simulink model "onOff"  (R2013b)
settings: Solver=FixedStepDiscrete  SolverMode=SingleTasking  StartTime=0.0  StopTime=10.0  FixedStep=0.01  RelTol=1e-3
undefined symbols (not defined in the file or in its folder): JA1, JB1, JC1, nexys2iroobo_lib
libraries: xbsIndex_r4 x84
settings Model: Creator=laca  LastModifiedBy=laca
settings DebuggingCC: MultiTaskDSMMsg=warning  MultiTaskCondExecSysMsg=none  FcnCallInpInsideContextMsg=EnableAllAsWarning  StrictBusMsg=None
settings RTWCC: IncludeERTFirstTime=on

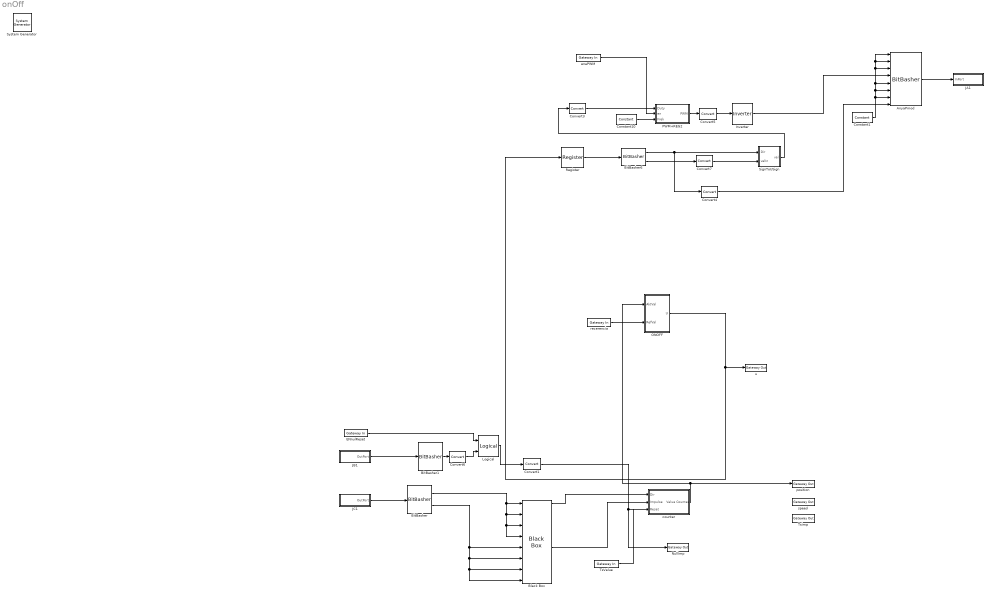
== system onOff ==
  " System Generator" : xbsIndex_r4/ System Generator  Tag=genX  xilinxfamily=spartan3e  part=xc3s1200e  speed=-4  package=fg320  synthesis_tool=XST  clock_wrapper=Clock Enables  directory=./netlist  proj_type=Project Navigator  Synth_file=XST Defaults  Impl_file=ISE Defaults  testbench=off  simulink_period=1  sysclk_period=20  dcm_input_clock_period=10  incr_netlist=off  trim_vbits=Everywhere in SubSystem  dbl_ovrd=According to Block Masks  core_generation=According to Block Masks  run_coregen=off  deprecated_control=off  eval_field=0  block_type=sysgen
  AnyaPmod : xbsIndex_r4/BitBasher  bitexpr=|  display_expr=off  sr_1=1  arith_type1=Unsigned  bin_pt1=0  sr_2=2  arith_type2=Unsigned  bin_pt2=0  sr_3=3  arith_type3=Unsigned  bin_pt3=0  sr_4=4  arith_type4=Unsigned  bin_pt4=0  dbl_ovrd=off  block_type=bitbasher
      | <!DOCTYPE HTML PUBLIC "-//W3C//DTD HTML 4.0//EN" "http://www.w3.org/TR/REC-html40/strict.dtd">
      | <html><head><meta name="qrichtext" content="1" /><style type="text/css">
      | p, li { white-space: pre-wrap; }
      | </style></head><body style=" font-family:'MS Shell Dlg 2'; font-size:8.25pt; font-weight:400; font-style:normal;">
      | <p style=" margin-top:12px; margin-bottom:12px; margin-left:0px; margin-right:0px; -qt-block-indent:0; text-indent:0px;"><span style=" font-family:'MS Shell Dlg'; font-size:8pt;">a={a8,a7,a6,a5,a4,a3,a2,a1}</span></p></body></html>
  BitBasher : xbsIndex_r4/BitBasher  bitexpr=|  display_expr=off  sr_1=1  arith_type1=Unsigned  bin_pt1=0  sr_2=2  arith_type2=Unsigned  bin_pt2=0  sr_3=3  arith_type3=Unsigned  bin_pt3=0  sr_4=4  arith_type4=Unsigned  bin_pt4=0  dbl_ovrd=off  block_type=bitbasher
      | <!DOCTYPE HTML PUBLIC "-//W3C//DTD HTML 4.0//EN" "http://www.w3.org/TR/REC-html40/strict.dtd">
      | <html><head><meta name="qrichtext" content="1" /><style type="text/css">
      | p, li { white-space: pre-wrap; }
      | </style></head><body style=" font-family:'MS Shell Dlg 2'; font-size:8.25pt; font-weight:400; font-style:normal;">
      | <p style=" margin-top:12px; margin-bottom:12px; margin-left:0px; margin-right:0px; -qt-block-indent:0; text-indent:0px;"><span style=" font-family:'MS Shell Dlg'; font-size:8pt;">A={a[0]}<br />B={a[1]}</span></p></body></html>
  BitBasher1 : xbsIndex_r4/BitBasher  bitexpr=|  display_expr=off  sr_1=1  arith_type1=Unsigned  bin_pt1=0  sr_2=2  arith_type2=Unsigned  bin_pt2=0  sr_3=3  arith_type3=Unsigned  bin_pt3=0  sr_4=4  arith_type4=Unsigned  bin_pt4=0  dbl_ovrd=off  block_type=bitbasher
      | <!DOCTYPE HTML PUBLIC "-//W3C//DTD HTML 4.0//EN" "http://www.w3.org/TR/REC-html40/strict.dtd">
      | <html><head><meta name="qrichtext" content="1" /><style type="text/css">
      | p, li { white-space: pre-wrap; }
      | </style></head><body style=" font-family:'MS Shell Dlg 2'; font-size:8.25pt; font-weight:400; font-style:normal;">
      | <p style=" margin-top:12px; margin-bottom:12px; margin-left:0px; margin-right:0px; -qt-block-indent:0; text-indent:0px;"><span style=" font-family:'MS Shell Dlg'; font-size:8pt;">Ar={ar[0]}<br /></span></p></body></html>
  BitBasher6 : xbsIndex_r4/BitBasher  bitexpr=|  display_expr=off  sr_1=1  arith_type1=Unsigned  bin_pt1=0  sr_2=2  arith_type2=Unsigned  bin_pt2=0  sr_3=3  arith_type3=Unsigned  bin_pt3=0  sr_4=4  arith_type4=Unsigned  bin_pt4=0  dbl_ovrd=off  block_type=bitbasher
      | <!DOCTYPE HTML PUBLIC "-//W3C//DTD HTML 4.0//EN" "http://www.w3.org/TR/REC-html40/strict.dtd">
      | <html><head><meta name="qrichtext" content="1" /><style type="text/css">
      | p, li { white-space: pre-wrap; }
      | </style></head><body style=" font-family:'MS Shell Dlg 2'; font-size:8.25pt; font-weight:400; font-style:normal;">
      | <p style=" margin-top:12px; margin-bottom:12px; margin-left:0px; margin-right:0px; -qt-block-indent:0; text-indent:0px;"><span style=" font-family:'MS Shell Dlg'; font-size:8pt;">dir={a[16]}<br />val={a[15:0]}</span></p></body></html>
  Black Box : xbsIndex_r4/Black Box  init_code=top_level_config  sim_method=ISE Simulator  verbose=off  block_type=blackbox2
  Constant1 : xbsIndex_r4/Constant  const=1  gui_display_data_type=Boolean  arith_type=Boolean  n_bits=16  bin_pt=0  preci_type=Single  exp_width=8  frac_width=24  explicit_period=on  period=1  equ=P=C  opselect=C  inp2=PCIN>>17  opr=+  inp1=P  carry=CIN  dbl_ovrd=off  block_type=constant
  Constant10 : xbsIndex_r4/Constant  const=65535  gui_display_data_type=Fixed-point  arith_type=Unsigned  n_bits=16  bin_pt=0  preci_type=Single  exp_width=8  frac_width=24  explicit_period=on  period=1  equ=P=C  opselect=C  inp2=PCIN>>17  opr=+  inp1=P  carry=CIN  dbl_ovrd=off  block_type=constant
  Convert1 : xbsIndex_r4/Convert  gui_display_data_type=Fixed-point  arith_type=Unsigned  n_bits=1  bin_pt=0  float_type=Single  exp_bits=8  fraction_bits=24  quantization=Truncate  overflow=Wrap  en=off  latency=0  dbl_ovrd=off  pipeline=off  block_type=convert
  Convert3 : xbsIndex_r4/Convert  gui_display_data_type=Fixed-point  arith_type=Unsigned  n_bits=16  bin_pt=0  float_type=Single  exp_bits=8  fraction_bits=24  quantization=Truncate  overflow=Wrap  en=off  latency=0  dbl_ovrd=off  pipeline=off  block_type=convert
  Convert4 : xbsIndex_r4/Convert  gui_display_data_type=Boolean  arith_type=Boolean  n_bits=17  bin_pt=0  float_type=Single  exp_bits=8  fraction_bits=24  quantization=Truncate  overflow=Wrap  en=off  latency=0  dbl_ovrd=off  pipeline=off  block_type=convert
  Convert5 : xbsIndex_r4/Convert  gui_display_data_type=Boolean  arith_type=Boolean  n_bits=17  bin_pt=0  float_type=Single  exp_bits=8  fraction_bits=24  quantization=Truncate  overflow=Wrap  en=off  latency=0  dbl_ovrd=off  pipeline=off  block_type=convert
  Convert6 : xbsIndex_r4/Convert  gui_display_data_type=Boolean  arith_type=Boolean  n_bits=17  bin_pt=0  float_type=Single  exp_bits=8  fraction_bits=24  quantization=Truncate  overflow=Wrap  en=off  latency=0  dbl_ovrd=off  pipeline=off  block_type=convert
  Convert7 : xbsIndex_r4/Convert  gui_display_data_type=Fixed-point  arith_type=Unsigned  n_bits=16  bin_pt=0  float_type=Single  exp_bits=8  fraction_bits=24  quantization=Truncate  overflow=Wrap  en=off  latency=0  dbl_ovrd=off  pipeline=off  block_type=convert
  ENnulReset : xbsIndex_r4/Gateway In  gui_display_data_type=Boolean  arith_type=Boolean  n_bits=17  bin_pt=0  preci_type=Single  exp_width=8  frac_width=24  quantization="Round  (unbiased: +/- Inf)"  overflow=Saturate  period=1  dbl_ovrd=off  timing_constraint=None  locs_specified=off  LOCs={}  UseAsADC=off  ADCChannel='1'  inherit_from_input=off  hdl_port=on  block_type=gatewayin
  Inverter : xbsIndex_r4/Inverter  en=off  latency=0  dbl_ovrd=off  block_type=inv
  JA1 : Subsystem  AncestorBlock=nexys2iroobo_lib/JA1  mask(Non-Memory-Mapped Output Port){show_out=off}
      mask prompts: show_out "Provide Output Double"
      mask help:
      | Port Name: "JA1"
      | Port Type: 8-bit Vector
      mask init:
      | [bg,fg] = xlcmap('IO',0);
      | iPos = get_param(gcb,'Position');
      | iWidth=iPos(3)-iPos(1);
      | iHeight=iPos(4)-iPos(2);
      | [logoX, logoY] = xlogo(iPos);
      | if (show_out)
      |     old = find_system(gcb, 'LookUnderMasks', 'all', 'Name', 'Terminator');
      |     if (length(old) > 0)
      |         replace_block(gcb, 'Name', 'Terminator', 'OutPort', 'noprompt');
      |         set_param([gcb '/Terminator'], 'Name', 'OutPort');
      |     end
      |     portdir = 'output';
      |     portstr = 'dbl';
      | else
      |     old = find_system(gcb, 'LookUnderMasks', 'all', 'name', 'OutPort');
      |     if (length(old) > 0)
      |         replace_block(gcb, 'Name', 'OutPort', 'Terminator', 'noprompt');
      |         set_param([gcb '/OutPort'], 'Name', 'Terminator');
      |     end
      |     portdir = 'input';
      |     portstr = '';
      | end
      settings: CopyFcn=set_param(gcb,'LinkStatus','inactive');
      mask Display:
      | patch([0 iWidth iWidth 0],[0 0 iHeight iHeight] , bg);
      | patch(logoX,logoY, fg);
      | plot([0 0 iWidth iWidth 0], [0 iHeight iHeight 0 0]);
      | port_label(portdir,1,portstr);
      | port_label('input',1,'JA1');
      | text(iWidth-10,5,'nmm');
  JB1 : Subsystem  AncestorBlock=nexys2iroobo_lib/JB1  mask(Non-Memory-Mapped Input Port){signed=off, bpt=0, show_in=off, c=0}
      mask prompts: signed "Signed  (2's comp)"; bpt "Binary Point"; show_in "Provide Input Double"; c "Constant for Simulation"
      mask help:
      | Port Name: "JB1"
      | Port Type: 8-bit Vector
      mask init:
      | [bg,fg] = xlcmap('IO',0);
      | iPos = get_param(gcb,'Position');
      | iWidth=iPos(3)-iPos(1);
      | iHeight=iPos(4)-iPos(2);
      | [logoX, logoY] = xlogo(iPos);
      | if (signed)
      |     set_param([gcb '/JB1'],'arith_type','Signed  (2''s comp)');
      | else
      |     set_param([gcb '/JB1'],'arith_type','Unsigned');
      | end
      | if (show_in)
      |     old = find_system(gcb, 'LookUnderMasks', 'all', 'Name', 'Constant');
      |     if (length(old) > 0)
      |         replace_block(gcb, 'Name', 'Constant', 'InPort', 'noprompt');
      |         set_param([gcb '/Constant'], 'Name', 'InPort');
      |     end
      |     portdir = 'input';
      |     portstr = 'dbl';
      | else
      |     old = find_system(gcb, 'LookUnderMasks', 'all', 'Name', 'InPort');
      |     if (length(old) > 0)
      |         replace_block(gcb, 'Name', 'InPort', 'Constant', 'noprompt');
      |         set_param([gcb '/InPort'], 'Name', 'Constant');
      |         set_param([gcb '/Constant'], 'Value', 'c');
      |     end
      |     portdir = 'output';
      |     portstr = '';
      | end
      settings: CopyFcn=set_param(gcb,'LinkStatus','inactive');
      mask Callback show_in:
      | mask_vis = get_param(gcb, 'MaskVisibilities');
      | if (strcmp(get_param(gcb, 'show_in'),'on'))
      |     mask_vis(4) = {'off'};
      | else
      |     mask_vis(4) = {'on'};
      | end
      | set_param(gcb, 'MaskVisibilities', mask_vis);
      mask Display:
      | patch([0 iWidth iWidth 0],[0 0 iHeight iHeight] , bg);
      | patch(logoX,logoY, fg);
      | plot([0 0 iWidth iWidth 0], [0 iHeight iHeight 0 0]);
      | port_label(portdir,1,portstr);
      | port_label('output',1,'JB1');
      | text(2,5,'nmm');
  JC1 : Subsystem  AncestorBlock=nexys2iroobo_lib/JC1  mask(Non-Memory-Mapped Input Port){signed=off, bpt=0, show_in=off, c=0}
      mask prompts: signed "Signed  (2's comp)"; bpt "Binary Point"; show_in "Provide Input Double"; c "Constant for Simulation"
      mask help:
      | Port Name: "JC1"
      | Port Type: 8-bit Vector
      mask init:
      | [bg,fg] = xlcmap('IO',0);
      | iPos = get_param(gcb,'Position');
      | iWidth=iPos(3)-iPos(1);
      | iHeight=iPos(4)-iPos(2);
      | [logoX, logoY] = xlogo(iPos);
      | if (signed)
      |     set_param([gcb '/JC1'],'arith_type','Signed  (2''s comp)');
      | else
      |     set_param([gcb '/JC1'],'arith_type','Unsigned');
      | end
      | if (show_in)
      |     old = find_system(gcb, 'LookUnderMasks', 'all', 'Name', 'Constant');
      |     if (length(old) > 0)
      |         replace_block(gcb, 'Name', 'Constant', 'InPort', 'noprompt');
      |         set_param([gcb '/Constant'], 'Name', 'InPort');
      |     end
      |     portdir = 'input';
      |     portstr = 'dbl';
      | else
      |     old = find_system(gcb, 'LookUnderMasks', 'all', 'Name', 'InPort');
      |     if (length(old) > 0)
      |         replace_block(gcb, 'Name', 'InPort', 'Constant', 'noprompt');
      |         set_param([gcb '/InPort'], 'Name', 'Constant');
      |         set_param([gcb '/Constant'], 'Value', 'c');
      |     end
      |     portdir = 'output';
      |     portstr = '';
      | end
      settings: CopyFcn=set_param(gcb,'LinkStatus','inactive');
      mask Callback show_in:
      | mask_vis = get_param(gcb, 'MaskVisibilities');
      | if (strcmp(get_param(gcb, 'show_in'),'on'))
      |     mask_vis(4) = {'off'};
      | else
      |     mask_vis(4) = {'on'};
      | end
      | set_param(gcb, 'MaskVisibilities', mask_vis);
      mask Display:
      | patch([0 iWidth iWidth 0],[0 0 iHeight iHeight] , bg);
      | patch(logoX,logoY, fg);
      | plot([0 0 iWidth iWidth 0], [0 iHeight iHeight 0 0]);
      | port_label(portdir,1,portstr);
      | port_label('output',1,'JC1');
      | text(2,5,'nmm');
  Logical : xbsIndex_r4/Logical  logical_function=AND  inputs=2  en=off  latency=0  precision=User Defined  arith_type="Signed  (2's comp)"  n_bits=1  bin_pt=0  align_bp=on  dbl_ovrd=off  block_type=logical
  NullImp : xbsIndex_r4/Gateway Out  inherit_from_input=off  hdl_port=on  timing_constraint=None  locs_specified=off  LOCs={}  UseAsDAC=off  DACChannel='1'  block_type=gatewayout
  ONOFF : Subsystem
  PWM+REG2 : Subsystem
  Register : xbsIndex_r4/Register  init=0  rst=off  en=off  dbl_ovrd=off  block_type=register
  SignToUSign : Subsystem
  TsValue : xbsIndex_r4/Gateway In  gui_display_data_type=Fixed-point  arith_type=Unsigned  n_bits=24  bin_pt=0  preci_type=Single  exp_width=8  frac_width=24  quantization="Round  (unbiased: +/- Inf)"  overflow=Saturate  period=1  dbl_ovrd=off  timing_constraint=None  locs_specified=off  LOCs={}  UseAsADC=off  ADCChannel='1'  inherit_from_input=off  hdl_port=on  block_type=gatewayin
  Tsimp : xbsIndex_r4/Gateway Out  inherit_from_input=off  hdl_port=on  timing_constraint=None  locs_specified=off  LOCs={}  UseAsDAC=off  DACChannel='1'  block_type=gatewayout
  counter : Subsystem
  enaPWM : xbsIndex_r4/Gateway In  gui_display_data_type=Boolean  arith_type=Boolean  n_bits=32  bin_pt=0  preci_type=Single  exp_width=8  frac_width=24  quantization="Round  (unbiased: +/- Inf)"  overflow=Saturate  period=1  dbl_ovrd=off  timing_constraint=None  locs_specified=off  LOCs={}  UseAsADC=off  ADCChannel='1'  inherit_from_input=off  hdl_port=on  block_type=gatewayin
  position : xbsIndex_r4/Gateway Out  inherit_from_input=off  hdl_port=on  timing_constraint=None  locs_specified=off  LOCs={}  UseAsDAC=off  DACChannel='1'  block_type=gatewayout
  recerencia : xbsIndex_r4/Gateway In  gui_display_data_type=Fixed-point  arith_type="Signed  (2's comp)"  n_bits=16  bin_pt=0  preci_type=Single  exp_width=8  frac_width=24  quantization="Round  (unbiased: +/- Inf)"  overflow=Saturate  period=1  dbl_ovrd=off  timing_constraint=None  locs_specified=off  LOCs={}  UseAsADC=off  ADCChannel='1'  inherit_from_input=off  hdl_port=on  block_type=gatewayin
  speed : xbsIndex_r4/Gateway Out  inherit_from_input=off  hdl_port=on  timing_constraint=None  locs_specified=off  LOCs={}  UseAsDAC=off  DACChannel='1'  block_type=gatewayout
  u : xbsIndex_r4/Gateway Out  inherit_from_input=off  hdl_port=on  timing_constraint=None  locs_specified=off  LOCs={}  UseAsDAC=off  DACChannel='1'  block_type=gatewayout
  wires:
  Constant10/1 -> PWM+REG2/3(Frek)
  enaPWM/1 -> PWM+REG2/2(en)
  PWM+REG2/1(PWM) -> Convert5/1
  BitBasher6/1 -> Convert4/1, SignToUSign/1(Dir)
  BitBasher6/2 -> Convert7/1
  SignToUSign/1(val) -> Convert3/1
  Inverter/1 -> AnyaPmod/4
  ONOFF/1(U) -> Register/1, u/1
  Convert3/1 -> PWM+REG2/1(Duty)
  Convert4/1 -> AnyaPmod/8
  Convert5/1 -> Inverter/1
  Convert7/1 -> SignToUSign/2(valIn)
  Register/1 -> BitBasher6/1
  AnyaPmod/1 -> JA1/1(InPort)
  Constant1/1 -> AnyaPmod/3, AnyaPmod/2, AnyaPmod/1, AnyaPmod/5, AnyaPmod/6, AnyaPmod/7
  Black Box/1 -> counter/1(Dir)
  Black Box/5 -> counter/2(Impulse)
  JC1/1(OutPort) -> BitBasher/1
  BitBasher/1 -> Black Box/4, Black Box/3, Black Box/2, Black Box/1
  BitBasher/2 -> Black Box/5, Black Box/6, Black Box/7, Black Box/8
  counter/1(Value Counter) -> ONOFF/1(AktVal), position/1
  TsValue/1 -> ?
  ? -> speed/1
  JB1/1(OutPort) -> BitBasher1/1
  Logical/1 -> Convert1/1
  ? -> Tsimp/1
  BitBasher1/1 -> Convert6/1
  ENnulReset/1 -> Logical/1
  Convert1/1 -> counter/3(Reset), NullImp/1
  Convert6/1 -> Logical/2
  recerencia/1 -> ONOFF/2(RefVal)

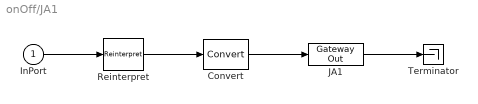
== system onOff/JA1 ==
  InPort : Inport
  Convert : xbsIndex_r4/Convert  gui_display_data_type=Fixed-point  arith_type=Unsigned  n_bits=8  bin_pt=0  float_type=Single  exp_bits=8  fraction_bits=24  quantization=Truncate  overflow=Wrap  en=off  latency=0  dbl_ovrd=off  pipeline=off  block_type=convert
  JA1 : xbsIndex_r4/Gateway Out  inherit_from_input=off  hdl_port=on  timing_constraint=None  locs_specified=on  LOCs={'M16','M14','L16','K13','M15','L17','K12','L15'}  UseAsDAC=off  DACChannel='1'  block_type=gatewayout
      settings: sginterface={'Xilinx'=>{'jtaghwcosim'=>{'non_memory_mapped_port'=>'JA1'}}}
  Reinterpret : xbsIndex_r4/Reinterpret  force_arith_type=off  arith_type=Unsigned  force_bin_pt=off  bin_pt=0  block_type=reinterpret
  Terminator : Terminator
  wires:
  JA1/1 -> Terminator/1
  Convert/1 -> JA1/1
  Reinterpret/1 -> Convert/1
  InPort/1 -> Reinterpret/1

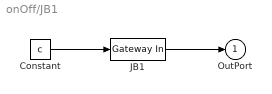
== system onOff/JB1 ==
  Constant : Constant  Value=c
  JB1 : xbsIndex_r4/Gateway In  gui_display_data_type=Fixed-point  arith_type=Unsigned  n_bits=8  bin_pt=max(0,min(bpt,8))  preci_type=Single  exp_width=8  frac_width=24  quantization="Round  (unbiased: +/- Inf)"  overflow=Saturate  period=1  dbl_ovrd=off  timing_constraint=None  locs_specified=on  LOCs={'U18','T18','R16','P17','T17','R15','R18','M13'}  UseAsADC=off  ADCChannel='1'  inherit_from_input=off  hdl_port=on  block_type=gatewayin
      settings: sginterface={'Xilinx'=>{'jtaghwcosim'=>{'non_memory_mapped_port'=>'JB1'}}}
  OutPort : Outport
  wires:
  Constant/1 -> JB1/1
  JB1/1 -> OutPort/1

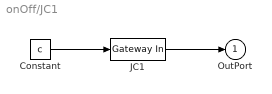
== system onOff/JC1 ==
  Constant : Constant  Value=c
  JC1 : xbsIndex_r4/Gateway In  gui_display_data_type=Fixed-point  arith_type=Unsigned  n_bits=8  bin_pt=max(0,min(bpt,8))  preci_type=Single  exp_width=8  frac_width=24  quantization="Round  (unbiased: +/- Inf)"  overflow=Saturate  period=1  dbl_ovrd=off  timing_constraint=None  locs_specified=on  LOCs={'J12','G16','F14','H15','H16','G13','J16','G15'}  UseAsADC=off  ADCChannel='1'  inherit_from_input=off  hdl_port=on  block_type=gatewayin
      settings: sginterface={'Xilinx'=>{'jtaghwcosim'=>{'non_memory_mapped_port'=>'JC1'}}}
  OutPort : Outport
  wires:
  Constant/1 -> JC1/1
  JC1/1 -> OutPort/1

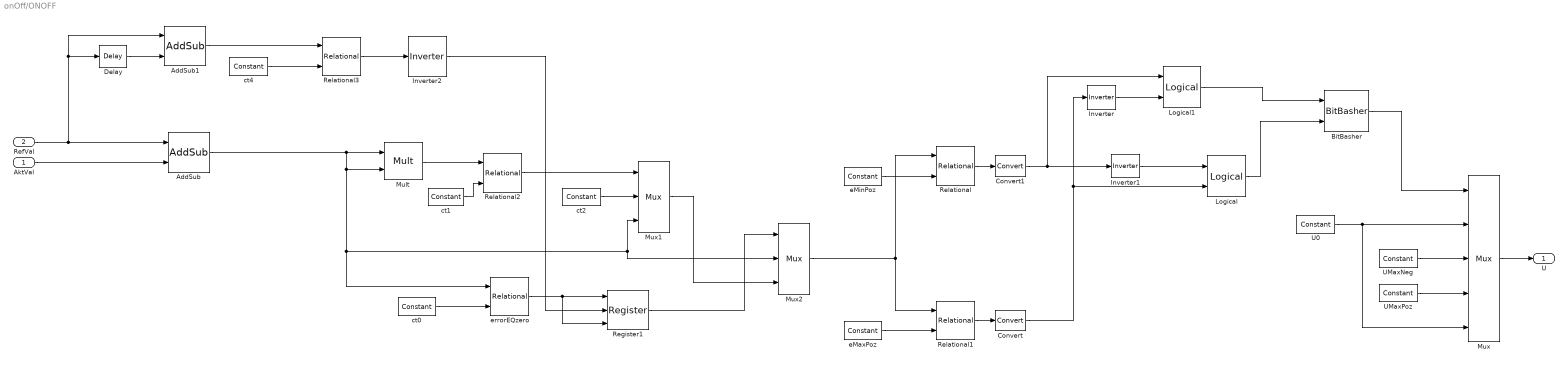
== system onOff/ONOFF ==
  AktVal : Inport
  RefVal : Inport  Port=2
  AddSub : xbsIndex_r4/AddSub  mode=Subtraction  use_carryin=off  use_carryout=off  en=off  latency=0  precision=User Defined  arith_type="Signed  (2's comp)"  n_bits=17  bin_pt=0  quantization=Truncate  overflow=Saturate  dbl_ovrd=off  use_behavioral_HDL=off  hw_selection=Fabric  pipelined=off  block_type=addsub
  AddSub1 : xbsIndex_r4/AddSub  mode=Subtraction  use_carryin=off  use_carryout=off  en=off  latency=0  precision=User Defined  arith_type="Signed  (2's comp)"  n_bits=17  bin_pt=0  quantization=Truncate  overflow=Wrap  dbl_ovrd=off  use_behavioral_HDL=off  hw_selection=Fabric  pipelined=off  block_type=addsub
  BitBasher : xbsIndex_r4/BitBasher  bitexpr=|  display_expr=off  sr_1=1  arith_type1=Unsigned  bin_pt1=0  sr_2=2  arith_type2=Unsigned  bin_pt2=0  sr_3=3  arith_type3=Unsigned  bin_pt3=0  sr_4=4  arith_type4=Unsigned  bin_pt4=0  dbl_ovrd=off  block_type=bitbasher
      | <!DOCTYPE HTML PUBLIC "-//W3C//DTD HTML 4.0//EN" "http://www.w3.org/TR/REC-html40/strict.dtd">
      | <html><head><meta name="qrichtext" content="1" /><style type="text/css">
      | p, li { white-space: pre-wrap; }
      | </style></head><body style=" font-family:'MS Shell Dlg 2'; font-size:8.25pt; font-weight:400; font-style:normal;">
      | <p style=" margin-top:12px; margin-bottom:12px; margin-left:0px; margin-right:0px; -qt-block-indent:0; text-indent:0px;"><span style=" font-family:'MS Shell Dlg'; font-size:8pt;">a={b,c}</span></p></body></html>
  Convert : xbsIndex_r4/Convert  gui_display_data_type=Boolean  arith_type=Boolean  n_bits=16  bin_pt=14  float_type=Single  exp_bits=8  fraction_bits=24  quantization=Truncate  overflow=Wrap  en=off  latency=0  dbl_ovrd=off  pipeline=off  block_type=convert
  Convert1 : xbsIndex_r4/Convert  gui_display_data_type=Boolean  arith_type=Boolean  n_bits=16  bin_pt=14  float_type=Single  exp_bits=8  fraction_bits=24  quantization=Truncate  overflow=Wrap  en=off  latency=0  dbl_ovrd=off  pipeline=off  block_type=convert
  Delay : xbsIndex_r4/Delay  rst=off  infoeditControl=Selection of Reset will increase slice count due to use of real FFs and instead of SRLs  en=off  latency=1  dbl_ovrd=off  reg_retiming=off  block_type=delay
  Inverter : xbsIndex_r4/Inverter  en=off  latency=0  dbl_ovrd=off  block_type=inv
  Inverter1 : xbsIndex_r4/Inverter  en=off  latency=0  dbl_ovrd=off  block_type=inv
  Inverter2 : xbsIndex_r4/Inverter  en=off  latency=0  dbl_ovrd=off  block_type=inv
  Logical : xbsIndex_r4/Logical  logical_function=AND  inputs=2  en=off  latency=0  precision=Full  arith_type=Unsigned  n_bits=16  bin_pt=0  align_bp=on  dbl_ovrd=off  block_type=logical
  Logical1 : xbsIndex_r4/Logical  logical_function=AND  inputs=2  en=off  latency=0  precision=Full  arith_type=Unsigned  n_bits=16  bin_pt=0  align_bp=on  dbl_ovrd=off  block_type=logical
  Mult : xbsIndex_r4/Mult  precision=User Defined  arith_type="Signed  (2's comp)"  n_bits=17  bin_pt=0  quantization=Truncate  overflow=Saturate  en=off  latency=3  dbl_ovrd=off  use_behavioral_HDL=off  opt=Speed  use_embedded=on  optimum_pipeline=off  pipeline=on  use_rpm=on  placement_style=Triangular  block_type=mult
  Mux : xbsIndex_r4/Mux  inputs=4  en=off  latency=0  precision=User Defined  arith_type="Signed  (2's comp)"  n_bits=17  bin_pt=0  quantization=Truncate  overflow=Wrap  dbl_ovrd=off  block_type=mux
  Mux1 : xbsIndex_r4/Mux  inputs=2  en=off  latency=0  precision=User Defined  arith_type="Signed  (2's comp)"  n_bits=17  bin_pt=0  quantization=Truncate  overflow=Wrap  dbl_ovrd=off  block_type=mux
  Mux2 : xbsIndex_r4/Mux  inputs=2  en=off  latency=0  precision=User Defined  arith_type="Signed  (2's comp)"  n_bits=17  bin_pt=0  quantization=Truncate  overflow=Wrap  dbl_ovrd=off  block_type=mux
  Register1 : xbsIndex_r4/Register  init=0  rst=on  en=on  dbl_ovrd=off  block_type=register
  Relational : xbsIndex_r4/Relational  mode=a>=b  en=off  latency=0  dbl_ovrd=off  block_type=relational
  Relational1 : xbsIndex_r4/Relational  mode=a<=b  en=off  latency=0  dbl_ovrd=off  block_type=relational
  Relational2 : xbsIndex_r4/Relational  mode=a>=b  en=off  latency=0  dbl_ovrd=off  block_type=relational
  Relational3 : xbsIndex_r4/Relational  mode=a=b  en=off  latency=0  dbl_ovrd=off  block_type=relational
  U0 : xbsIndex_r4/Constant  const=0  gui_display_data_type=Fixed-point  arith_type=Signed (2's comp)  n_bits=17  bin_pt=0  preci_type=Single  exp_width=8  frac_width=24  explicit_period=off  period=1  equ=P=C  opselect=C  inp2=PCIN>>17  opr=+  inp1=P  carry=CIN  dbl_ovrd=off  block_type=constant
  UMaxNeg : xbsIndex_r4/Constant  const=-65535  gui_display_data_type=Fixed-point  arith_type=Signed (2's comp)  n_bits=17  bin_pt=0  preci_type=Single  exp_width=8  frac_width=24  explicit_period=off  period=1  equ=P=C  opselect=C  inp2=PCIN>>17  opr=+  inp1=P  carry=CIN  dbl_ovrd=off  block_type=constant
  UMaxPoz : xbsIndex_r4/Constant  const=65535  gui_display_data_type=Fixed-point  arith_type=Signed (2's comp)  n_bits=17  bin_pt=0  preci_type=Single  exp_width=8  frac_width=24  explicit_period=off  period=1  equ=P=C  opselect=C  inp2=PCIN>>17  opr=+  inp1=P  carry=CIN  dbl_ovrd=off  block_type=constant
  ct0 : xbsIndex_r4/Constant  const=0  gui_display_data_type=Fixed-point  arith_type=Signed (2's comp)  n_bits=17  bin_pt=0  preci_type=Single  exp_width=8  frac_width=24  explicit_period=off  period=1  equ=P=C  opselect=C  inp2=PCIN>>17  opr=+  inp1=P  carry=CIN  dbl_ovrd=off  block_type=constant
  ct1 : xbsIndex_r4/Constant  const=3  gui_display_data_type=Fixed-point  arith_type=Signed (2's comp)  n_bits=17  bin_pt=0  preci_type=Single  exp_width=8  frac_width=24  explicit_period=off  period=1  equ=P=C  opselect=C  inp2=PCIN>>17  opr=+  inp1=P  carry=CIN  dbl_ovrd=off  block_type=constant
  ct2 : xbsIndex_r4/Constant  const=0  gui_display_data_type=Fixed-point  arith_type=Signed (2's comp)  n_bits=17  bin_pt=0  preci_type=Single  exp_width=8  frac_width=24  explicit_period=off  period=1  equ=P=C  opselect=C  inp2=PCIN>>17  opr=+  inp1=P  carry=CIN  dbl_ovrd=off  block_type=constant
  ct4 : xbsIndex_r4/Constant  const=0  gui_display_data_type=Fixed-point  arith_type=Signed (2's comp)  n_bits=17  bin_pt=0  preci_type=Single  exp_width=8  frac_width=24  explicit_period=off  period=1  equ=P=C  opselect=C  inp2=PCIN>>17  opr=+  inp1=P  carry=CIN  dbl_ovrd=off  block_type=constant
  eMaxPoz : xbsIndex_r4/Constant  const=-1  gui_display_data_type=Fixed-point  arith_type=Signed (2's comp)  n_bits=17  bin_pt=0  preci_type=Single  exp_width=8  frac_width=24  explicit_period=off  period=1  equ=P=C  opselect=C  inp2=PCIN>>17  opr=+  inp1=P  carry=CIN  dbl_ovrd=off  block_type=constant
  eMinPoz : xbsIndex_r4/Constant  const=1  gui_display_data_type=Fixed-point  arith_type=Signed (2's comp)  n_bits=17  bin_pt=0  preci_type=Single  exp_width=8  frac_width=24  explicit_period=off  period=1  equ=P=C  opselect=C  inp2=PCIN>>17  opr=+  inp1=P  carry=CIN  dbl_ovrd=off  block_type=constant
  errorEQzero : xbsIndex_r4/Relational  mode=a=b  en=off  latency=0  dbl_ovrd=off  block_type=relational
  U : Outport
  wires:
  Mux/1 -> U/1
  UMaxNeg/1 -> Mux/3
  eMinPoz/1 -> Relational/2
  AddSub/1 -> Mult/2, errorEQzero/1, Mux1/3, Mux2/2, Mult/1
  eMaxPoz/1 -> Relational1/2
  Relational/1 -> Convert1/1
  Relational1/1 -> Convert/1
  Logical/1 -> BitBasher/2
  Convert/1 -> Logical/2, Inverter/1
  Convert1/1 -> Inverter1/1, Logical1/1
  BitBasher/1 -> Mux/1
  Inverter/1 -> Logical1/2
  Inverter1/1 -> Logical/1
  Logical1/1 -> BitBasher/1
  UMaxPoz/1 -> Mux/4
  U0/1 -> Mux/5, Mux/2
  Relational2/1 -> Mux1/1
  Mult/1 -> Relational2/1
  ct1/1 -> Relational2/2
  ct2/1 -> Mux1/2
  Mux2/1 -> Relational/1, Relational1/1
  ct0/1 -> errorEQzero/2
  errorEQzero/1 -> Register1/1, Register1/3
  Mux1/1 -> Mux2/3
  Register1/1 -> Mux2/1
  RefVal/1 -> AddSub/1, AddSub1/1, Delay/1
  ct4/1 -> Relational3/2
  Delay/1 -> AddSub1/2
  AddSub1/1 -> Relational3/1
  Relational3/1 -> Inverter2/1
  Inverter2/1 -> Register1/2
  AktVal/1 -> AddSub/2

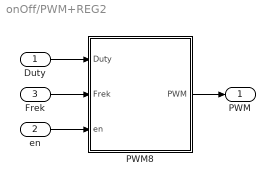
== system onOff/PWM+REG2 ==
  Duty : Inport
  en : Inport  Port=2
  Frek : Inport  Port=3
  PWM8 : Subsystem
  PWM : Outport
  wires:
  Duty/1 -> PWM8/1(Duty)
  en/1 -> PWM8/3(en)
  PWM8/1(PWM) -> PWM/1
  Frek/1 -> PWM8/2(Frek)

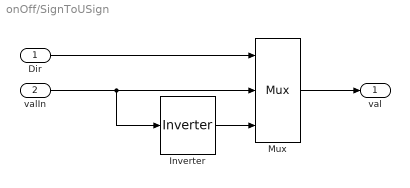
== system onOff/SignToUSign ==
  Dir : Inport
  valIn : Inport  Port=2
  Inverter : xbsIndex_r4/Inverter  en=off  latency=0  dbl_ovrd=off  block_type=inv
  Mux : xbsIndex_r4/Mux  inputs=2  en=off  latency=0  precision=User Defined  arith_type=Unsigned  n_bits=16  bin_pt=0  quantization=Truncate  overflow=Wrap  dbl_ovrd=off  block_type=mux
  val : Outport
  wires:
  Dir/1 -> Mux/1
  valIn/1 -> Inverter/1, Mux/2
  Mux/1 -> val/1
  Inverter/1 -> Mux/3

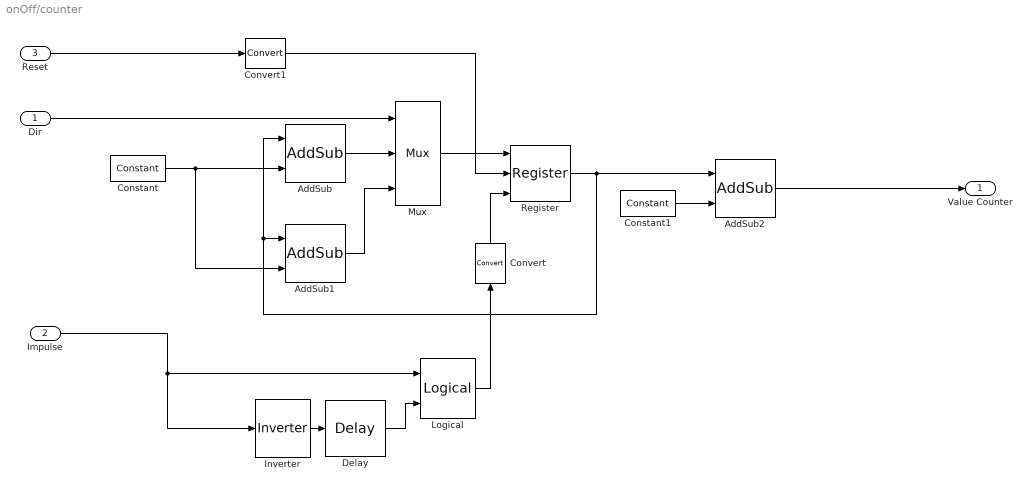
== system onOff/counter ==
  Dir : Inport
  Impulse : Inport  Port=2
  Reset : Inport  Port=3
  AddSub : xbsIndex_r4/AddSub  mode=Addition  use_carryin=off  use_carryout=off  en=off  latency=0  precision=Full  arith_type=Unsigned  n_bits=16  bin_pt=14  quantization=Truncate  overflow=Wrap  dbl_ovrd=off  use_behavioral_HDL=off  hw_selection=Fabric  pipelined=off  block_type=addsub
  AddSub1 : xbsIndex_r4/AddSub  mode=Subtraction  use_carryin=off  use_carryout=off  en=off  latency=0  precision=Full  arith_type=Unsigned  n_bits=16  bin_pt=14  quantization=Truncate  overflow=Wrap  dbl_ovrd=off  use_behavioral_HDL=off  hw_selection=Fabric  pipelined=off  block_type=addsub
  AddSub2 : xbsIndex_r4/AddSub  mode=Subtraction  use_carryin=off  use_carryout=off  en=off  latency=0  precision=User Defined  arith_type="Signed  (2's comp)"  n_bits=16  bin_pt=0  quantization=Truncate  overflow=Wrap  dbl_ovrd=off  use_behavioral_HDL=off  hw_selection=Fabric  pipelined=off  block_type=addsub
  Constant : xbsIndex_r4/Constant  const=1  gui_display_data_type=Fixed-point  arith_type=Unsigned  n_bits=16  bin_pt=0  preci_type=Single  exp_width=8  frac_width=24  explicit_period=off  period=1  equ=P=C  opselect=C  inp2=PCIN>>17  opr=+  inp1=P  carry=CIN  dbl_ovrd=off  block_type=constant
  Constant1 : xbsIndex_r4/Constant  const=32767+180  gui_display_data_type=Fixed-point  arith_type=Unsigned  n_bits=16  bin_pt=0  preci_type=Single  exp_width=8  frac_width=24  explicit_period=off  period=1  equ=P=C  opselect=C  inp2=PCIN>>17  opr=+  inp1=P  carry=CIN  dbl_ovrd=off  block_type=constant
  Convert : xbsIndex_r4/Convert  gui_display_data_type=Boolean  arith_type=Boolean  n_bits=16  bin_pt=14  float_type=Single  exp_bits=8  fraction_bits=24  quantization=Truncate  overflow=Wrap  en=off  latency=0  dbl_ovrd=off  pipeline=off  block_type=convert
  Convert1 : xbsIndex_r4/Convert  gui_display_data_type=Boolean  arith_type=Boolean  n_bits=16  bin_pt=14  float_type=Single  exp_bits=8  fraction_bits=24  quantization=Truncate  overflow=Wrap  en=off  latency=0  dbl_ovrd=off  pipeline=off  block_type=convert
  Delay : xbsIndex_r4/Delay  rst=off  infoeditControl=Selection of Reset will increase slice count due to use of real FFs and instead of SRLs  en=off  latency=1  dbl_ovrd=off  reg_retiming=off  block_type=delay
  Inverter : xbsIndex_r4/Inverter  en=off  latency=0  dbl_ovrd=off  block_type=inv
  Logical : xbsIndex_r4/Logical  logical_function=AND  inputs=2  en=off  latency=0  precision=Full  arith_type=Unsigned  n_bits=16  bin_pt=0  align_bp=on  dbl_ovrd=off  block_type=logical
  Mux : xbsIndex_r4/Mux  inputs=2  en=off  latency=0  precision=User Defined  arith_type=Unsigned  n_bits=16  bin_pt=0  quantization=Truncate  overflow=Wrap  dbl_ovrd=off  block_type=mux
  Register : xbsIndex_r4/Register  init=32767  rst=on  en=on  dbl_ovrd=off  block_type=register
  Value Counter : Outport
  wires:
  Mux/1 -> Register/1
  AddSub/1 -> Mux/2
  AddSub1/1 -> Mux/3
  Constant/1 -> AddSub/2, AddSub1/2
  Register/1 -> AddSub2/1, AddSub/1, AddSub1/1
  Dir/1 -> Mux/1
  Inverter/1 -> Delay/1
  Delay/1 -> Logical/2
  Logical/1 -> Convert/1
  Impulse/1 -> Logical/1, Inverter/1
  Constant1/1 -> AddSub2/2
  AddSub2/1 -> Value Counter/1
  Reset/1 -> Convert1/1
  Convert/1 -> Register/3
  Convert1/1 -> Register/2

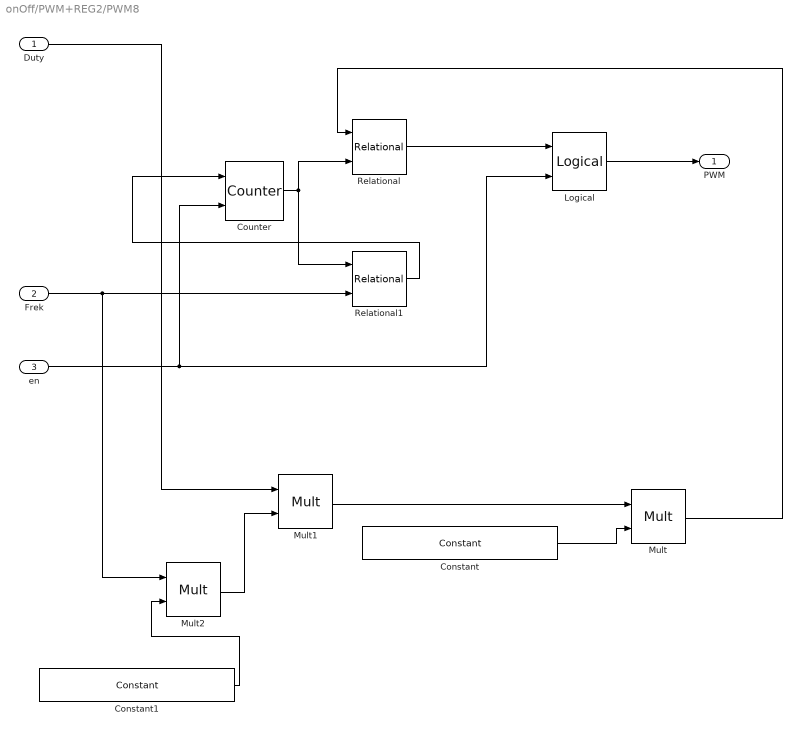
== system onOff/PWM+REG2/PWM8 ==
  Duty : Inport
  Frek : Inport  Port=2
  en : Inport  Port=3
  Constant : xbsIndex_r4/Constant  const=1/65535  gui_display_data_type=Fixed-point  arith_type=Signed (2's comp)  n_bits=32  bin_pt=20  preci_type=Single  exp_width=8  frac_width=24  explicit_period=off  period=1  equ=P=C  opselect=C  inp2=PCIN>>17  opr=+  inp1=P  carry=CIN  dbl_ovrd=off  block_type=constant
  Constant1 : xbsIndex_r4/Constant  const=0.95  gui_display_data_type=Fixed-point  arith_type=Signed (2's comp)  n_bits=16  bin_pt=14  preci_type=Single  exp_width=8  frac_width=24  explicit_period=off  period=1  equ=P=C  opselect=C  inp2=PCIN>>17  opr=+  inp1=P  carry=CIN  dbl_ovrd=off  block_type=constant
  Counter : xbsIndex_r4/Counter  cnt_type=Free Running  cnt_to=Inf  operation=Up  start_count=0  cnt_by_val=1  arith_type=Unsigned  n_bits=16  bin_pt=0  load_pin=off  rst=on  en=on  explicit_period=off  period=2*10^-2  dbl_ovrd=off  use_behavioral_HDL=off  implementation=Fabric  block_type=counter
  Logical : xbsIndex_r4/Logical  logical_function=AND  inputs=2  en=off  latency=0  precision=Full  arith_type=Unsigned  n_bits=16  bin_pt=0  align_bp=on  dbl_ovrd=off  block_type=logical
  Mult : xbsIndex_r4/Mult  precision=User Defined  arith_type=Unsigned  n_bits=16  bin_pt=0  quantization=Truncate  overflow=Saturate  en=off  latency=1  dbl_ovrd=off  use_behavioral_HDL=off  opt=Speed  use_embedded=on  optimum_pipeline=off  pipeline=on  use_rpm=on  placement_style=Triangular  block_type=mult
  Mult1 : xbsIndex_r4/Mult  precision=User Defined  arith_type=Unsigned  n_bits=32  bin_pt=0  quantization=Truncate  overflow=Saturate  en=off  latency=1  dbl_ovrd=off  use_behavioral_HDL=off  opt=Speed  use_embedded=on  optimum_pipeline=off  pipeline=on  use_rpm=on  placement_style=Triangular  block_type=mult
  Mult2 : xbsIndex_r4/Mult  precision=User Defined  arith_type=Unsigned  n_bits=16  bin_pt=0  quantization=Truncate  overflow=Saturate  en=off  latency=1  dbl_ovrd=off  use_behavioral_HDL=off  opt=Speed  use_embedded=on  optimum_pipeline=off  pipeline=on  use_rpm=on  placement_style=Triangular  block_type=mult
  Relational : xbsIndex_r4/Relational  mode=a>b  en=off  latency=0  dbl_ovrd=off  block_type=relational
  Relational1 : xbsIndex_r4/Relational  mode=a=b  en=off  latency=0  dbl_ovrd=off  block_type=relational
  PWM : Outport
  wires:
  Counter/1 -> Relational/2, Relational1/1
  Frek/1 -> Relational1/2, Mult2/1
  Relational1/1 -> Counter/1
  en/1 -> Logical/2, Counter/2
  Duty/1 -> Mult1/1
  Relational/1 -> Logical/1
  Logical/1 -> PWM/1
  Constant/1 -> Mult/2
  Mult1/1 -> Mult/1
  Mult/1 -> Relational/1
  Mult2/1 -> Mult1/2
  Constant1/1 -> Mult2/2
